simulink library "RespiratorCtrlLib"  (R2018b)
settings: Solver=VariableStepAuto  StartTime=0.0  StopTime=10.0  RelTol=1e-3
undefined symbols (not defined in the file or in its folder): AnalogMax, AnalogMin, aValveFullClose, aValveFullOpen, aValvePwm100, eSupervisorStates, fpDiffQAirInhalation, fpStatQAirInhalation, pDiffQAirAutoOffsetMax, pDiffQAirAutoOffsetMin, pDiffQAirAutoOffsetRateMax, pDiffQAirInhalationOffset, pDiffQAirScaledMax, pDiffQAirScaledMin, PressureMax, PressureMin, pStatQAirAutoOffsetMax, pStatQAirAutoOffsetMin, pStatQAirAutoOffsetRateMax, pStatQAirInhalationOffset, pStatQAirScaledMax, pStatQAirScaledMin, rPwmZeroDeg, VAnalogInputSpan, VpDiffQAirAnalogicDiagMax, VpDiffQAirAnalogicDiagMin, VpDiffQAirAnalogicMax, VpDiffQAirAnalogicMin, VpStatQAirAnalogicDiagMax, VpStatQAirAnalogicDiagMin, VpStatQAirAnalogicMax, VpStatQAirAnalogicMin
libraries: simulink x16, mbedblockslib x4, simulink_extras x2, $bdroot x2
(part 1 of 2)
settings Model: Creator=BRAUL  LastModifiedBy=VITIE

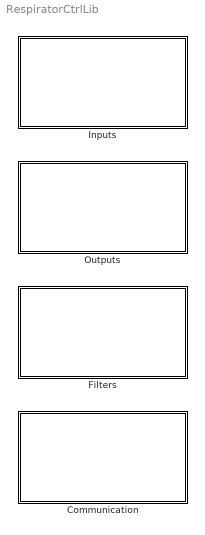
== system RespiratorCtrlLib ==
  Communication : Subsystem
  Filters : Subsystem
  Inputs : Subsystem
  Outputs : Subsystem

== system RespiratorCtrlLib/Communication ==
  Frame Multiplexer : Subsystem  TreatAsAtomicUnit=on  mask(CAN Frame multiplexer counter){MuxEndValue=1}
      mask prompts: MuxEndValue "Mutiplexer end value"
      mask help: Increase by one the output value at each sample time and reset the output (0) when previous value is equal to multiplexer end value
      settings: RTWSystemCode=Inline

== system RespiratorCtrlLib/Filters ==
  First order low pass : Subsystem  TreatAsAtomicUnit=on
      settings: RTWSystemCode=Inline
      mask Display: disp('1st Order\nLow pass')

== system RespiratorCtrlLib/Inputs ==
  Analogic Read : Subsystem  mask(Analogic Input Read){pinFunc=None, pinSelected=NC, TS=-1}
      mask prompts: pinFunc "Function"; pinSelected "Pin"; TS "Sample Time"
      mask help: Read the selected Nucleo STM32F411RE board pin as an analogic input
      mask init:
      | initAnalogicRead(gcb);
      settings: OpenFcn=|
      | setBlockPinNames(gcb);
      | open_system(gcb, 'mask');
      mask TypeOptions pinSelected: A0 | A1 | A2 | A3 | A4 | A5 | D0 | D1 | D2 | D3 | D4 | D5 | D6 | D7 | D8 | D9 | D10 | D11 | D12 | D13 | D14 | D15 | PA_0 | PA_1 | PA_2 | PA_3 | PA_4 | PA_5 | PA_6 | PA_7 | PA_8 | PA_9 | PA_10 | PA_11 | PA_12 | PA_13 | PA_14 | PA_15 | PB_0 | PB_1 | PB_2 | PB_3 | PB_4 | PB_5 | PB_6 | PB_7 | PB_8 | PB_9 | PB_10 | PB_11 | PB_12 | PB_13 | PB_14 | PB_15 | PC_0 | PC_1 | PC_2 | PC_3 | PC_4 | PC_5 | PC_6 | PC_7 | PC_8 | PC_9 | PC_10 | PC_11 | PC_12 | PC_13 | PC_14 | PC_15 | PD_2 | PH_0 | PH_1 | NC
      mask Display: disp('Analogic IN\nNone: NC')
  Button Processing : Subsystem  TreatAsAtomicUnit=on  mask(Push button debouncing){tDebounce=0.1, tSample=0.01, NDebounce=[]}
      mask prompts: tDebounce "Debounce time [sec]"; tSample "Sample time [sec]"
      mask help: Outputs the Pressed/Released state of the input push button according to user debouncing settings
      mask init:
      | % Compute debouncing sample count
      | if tSample > 0 && tDebounce > tSample
      |     
      |     NDebounce = tDebounce/tSample;
      |     
      |     maskDisplay = ['Push button\n' ...
      |                    'Debounce: ', ...
      |                    mat2str(tDebounce*1000), ...
      |                    ' ms'];
      |                
      |     set_param(gcb,'ForegroundColor', 'black');
      |     
      | else
      |     
      |     NDebounce = 2;
      |     
      |     warning([get_param(gcb, 'MaskType'), ...
      |              ' ', gcb, ' uses default debouncing setup ', ...
      |              mat2str(NDebounce), ' time steps']);
      |          
      |     maskDisplay = ['Push button\n' ...
      |                    'Debounce:\n', ...
      |                    mat2str(NDebounce), ...
      |                    ' time steps'];
      |                
      |     set_param(gcb,'ForegroundColor', 'orange');
      |     
      | end
      | 
      | % Update mask display
      | 
      | 
      | blkMask = Simulink.Mask.get(gcb);
      | blkMask.set('Display', ['disp(', char(39), maskDisplay, char(39), ')']);
      mask Display: disp('Push button\nDebounce: 100 ms')
  Differential Pressure Measurement : Subsystem  TreatAsAtomicUnit=on  mask(Differential pressure measurement){MeasName=Inhalation differential pressure, AnalogMin=VpDiffQAirAnalogicMin, AnalogMax=VpDiffQAirAnalogicMax, PressureMin=pDiffQAirScaledMin, PressureMax=pDiffQAirScaledMax, ZeroOffset=pDiffQAirInhalationOffset, CutOffFreq=fpDiffQAirInhalation, pOffsetMin=pDiffQAirAutoOffsetMin, pOffsetMax=pDiffQAirAutoOffsetMax, pOffsetRateMax=pDiffQAirAutoOffsetRateMax, VAnaMinDiag=VpDiffQAirAnalogicDiagMin, VAnaMaxDiag=VpDiffQAirAnalogicDiagMax}
      mask prompts: MeasName "Pressure name"; AnalogMin "Analogic value min [mV]"; AnalogMax "Analogic value max [mV]"; PressureMin "Pressure value min"; PressureMax "Pressure value max"; ZeroOffset "Static offset"; CutOffFreq "Filter cut-off frequency [Hz]"; pOffsetMin "Auto offset min"; pOffsetMax "Auto offset max"; pOffsetRateMax "Auto offset rate max"; VAnaMinDiag "Sensor diag analogic value min [mV]"; VAnaMaxDiag "Sensor diag analogic value max [mV]"
      mask help:
      | Convert and filter analog pressure input value to a physical measurement value using given linearization properties
      | Compute and apply a dynamic zero offset
      | Assert that sensor analogic value is contain within boundaries
      mask init:
      | % Update mask display
      | maskDisplay = [MeasName, '\nDifferential Pressure\nProcessing'];
      | 
      | blkMask = Simulink.Mask.get(gcb);
      | blkMask.set('Display', ['disp(', char(39), maskDisplay, char(39), ')']);
      mask DialogControl Container4 Prompt: ADC Conversion
      mask DialogControl Container7 Prompt: Filtering
      mask DialogControl Control3 Prompt: Pressure measurement 1st order low pass filter
      mask DialogControl Container8 Prompt: Auto Offset
      mask DialogControl Control4 Prompt: Pressure measurement dynamic auto offset
      mask DialogControl Container9 Prompt: Diagnostic
      mask DialogControl Control5 Prompt: Sensor analogic value diagnostic
      mask Display: disp('Inhalation differential pressure\nDifferential Pressure\nProcessing')
  Digital Read : Subsystem  mask(Digital Input Read){pinFunc=None, pinSelected=NC, TS=-1}
      mask prompts: pinFunc "Function"; pinSelected "Pin"; TS "Sample Time"
      mask help: Read the selected Nucleo STM32F411RE board pin as a digital input
      mask init:
      | initDigitalRead(gcb);
      settings: OpenFcn=|
      | setBlockPinNames(gcb);
      | open_system(gcb, 'mask');
      mask TypeOptions pinSelected: A0 | A1 | A2 | A3 | A4 | A5 | D0 | D1 | D2 | D3 | D4 | D5 | D6 | D7 | D8 | D9 | D10 | D11 | D12 | D13 | D14 | D15 | PA_0 | PA_1 | PA_2 | PA_3 | PA_4 | PA_5 | PA_6 | PA_7 | PA_8 | PA_9 | PA_10 | PA_11 | PA_12 | PA_13 | PA_14 | PA_15 | PB_0 | PB_1 | PB_2 | PB_3 | PB_4 | PB_5 | PB_6 | PB_7 | PB_8 | PB_9 | PB_10 | PB_11 | PB_12 | PB_13 | PB_14 | PB_15 | PC_0 | PC_1 | PC_2 | PC_3 | PC_4 | PC_5 | PC_6 | PC_7 | PC_8 | PC_9 | PC_10 | PC_11 | PC_12 | PC_13 | PC_14 | PC_15 | PD_2 | PH_0 | PH_1 | NC
      mask Display: disp('Digital IN\nNone: NC')
  Flow Computation : Subsystem  TreatAsAtomicUnit=on  mask(Flow measurement){measName=Flow, QRef=0, PStatRef=1, PDiffRef=1, kAlpha=0, kBeta=0}
      mask prompts: measName "Measurement name"; QRef "Reference flow [l/min]"; PStatRef "Reference static pressure [mbar]"; PDiffRef "Reference differential pressure [mbar]"; kAlpha "Alpha coefficient"; kBeta "Beta coefficient"
      mask help: Compute flow based on inputs static and differential pressure measurements using given parameters
      mask init:
      | % Update mask display
      | maskDisplay = [measName, '\nFlow'];
      | 
      | blkMask = Simulink.Mask.get(gcb);
      | blkMask.set('Display', ['disp(', char(39), maskDisplay, char(39), ')']);
      settings: RTWSystemCode=Inline
      mask Display: disp('Flow\nFlow')
  Input Scaling : Subsystem  TreatAsAtomicUnit=on  mask(Analog Input Scaling){inputName=MeasName, elecMin=AnalogMin, elecMax=AnalogMax, physicMin=PressureMin, physicMax=PressureMax, gain=0, offset=0}
      mask prompts: inputName "Measurement Name"; elecMin "Electrical range min [mV]"; elecMax "Electrical range max [mV]"; physicMin "Physical value min [SI]"; physicMax "Physical value max [SI]"
      mask help: Convert analog input value to a physical measurement value using given linearization properties
      mask init:
      | % Compute linearization gain & offset
      | gain = (physicMax - physicMin) / (elecMax - elecMin);
      | offset = physicMax - elecMax*gain;
      | 
      | % Update mask display
      | maskDisplay = [inputName, '\ninput\nscaling'];
      | 
      | blkMask = Simulink.Mask.get(gcb);
      | blkMask.set('Display', ['disp(', char(39), maskDisplay, char(39), ')']);
      settings: RTWSystemCode=Inline
      mask Display: disp('MeasName\ninput\nscaling')
  Static Pressure Measurement : Subsystem  TreatAsAtomicUnit=on  mask(Static pressure measurement){MeasName=Inhalation static pressure, AnalogMin=VpStatQAirAnalogicMin, AnalogMax=VpStatQAirAnalogicMax, PressureMin=pStatQAirScaledMin, PressureMax=pStatQAirScaledMax, ZeroOffset=pStatQAirInhalationOffset, CutOffFreq=fpStatQAirInhalation, VAnaMinDiag=VpStatQAirAnalogicDiagMin, VAnaMaxDiag=VpStatQAirAnalogicDiagMax}
      mask prompts: MeasName "Pressure name"; AnalogMin "Analogic value min [mV]"; AnalogMax "Analogic value max [mV]"; PressureMin "Pressure value min"; PressureMax "Pressure value max"; ZeroOffset "Static offset"; CutOffFreq "Filter cut-off frequency [Hz]"; VAnaMinDiag "Sensor diag analogic value min [mV]"; VAnaMaxDiag "Sensor diag analogic value max [mV]"
      mask help:
      | Convert and filter analog pressure input value to a physical measurement value using given linearization properties.
      | Apply a dynamic offset on the output pressure value.
      | Assert that sensor analogic value is contain within boundaries.
      mask init:
      | % Update mask display
      | maskDisplay = [MeasName, '\nStatic Pressure\nProcessing'];
      | 
      | blkMask = Simulink.Mask.get(gcb);
      | blkMask.set('Display', ['disp(', char(39), maskDisplay, char(39), ')']);
      mask DialogControl Container4 Prompt: ADC Conversion
      mask DialogControl Container7 Prompt: Filtering
      mask DialogControl Control3 Prompt: Pressure measurement 1st order low pass filter
      mask DialogControl Container9 Prompt: Diagnostic
      mask DialogControl Control5 Prompt: Sensor analogic value diagnostic
      mask Display: disp('Inhalation static pressure\nStatic Pressure\nProcessing')
  Static Pressures Offset : Subsystem  TreatAsAtomicUnit=on  mask(Static pressures offset computation){pOffsetMin=pStatQAirAutoOffsetMin, pOffsetMax=pStatQAirAutoOffsetMax, pOffsetRateMax=pStatQAirAutoOffsetRateMax}
      mask prompts: pOffsetMin "Auto offset min"; pOffsetMax "Auto offset max"; pOffsetRateMax "Auto offset rate max"
      mask help:
      | Compute pressure measurement dynamic offset of two static pressure measurements.
      | Offset is computed based on average value of inputs measurement in order to get both sensor on their mutual average value
      mask Display: disp('Static Pressures\nOffsets')
  User Setpoint : Subsystem  TreatAsAtomicUnit=on  mask(User setpoint){DefaultSetPoint=500, Increment=10, Decrement=10, MinSetPoint=300, MaxSetPoint=700}
      mask prompts: DefaultSetPoint "Default setpoint value"; Increment "Setpoint increment (on plus rising edge)"; Decrement "Setpoint decrement (on minus rising edge)"; MinSetPoint "Setpoint min value"; MaxSetPoint "Setpoint max value"
      mask help:
      | Output a user setpoint according to rising edge of 'Plus' and 'Minus' inputs.
      | When a rising edge of 'Plus' input is received, increment value is added to the previous setpoint.
      | When a rising edge of 'Minus' input is received, decrement value is substracted to the previous setpoint.
      | Final output value is saturated between setpoint min and max values.
      | When both 'Plus' and 'Minus' inputs are true at the same time, setpoint does not change.
      settings: RTWSystemCode=Inline
      mask Display:
      | port_label('input', 1, 'Plus')
      | port_label('input', 2, 'Minus')
      | port_label('output', 1, 'Setpoint')

== system RespiratorCtrlLib/Outputs ==
  Digital Write : Subsystem  mask(Digital Output Write){pinFunc=None, pinSelected=NC}
      mask prompts: pinFunc "Function"; pinSelected "Pin"
      mask help: Write the selected Nucleo STM32F411RE board pin as a digital output
      mask init:
      | initDigitalWrite(gcb);
      settings: OpenFcn=|
      | setBlockPinNames(gcb);
      | open_system(gcb, 'mask');
      mask TypeOptions pinSelected: A0 | A1 | A2 | A3 | A4 | A5 | D0 | D1 | D2 | D3 | D4 | D5 | D6 | D7 | D8 | D9 | D10 | D11 | D12 | D13 | D14 | D15 | PA_0 | PA_1 | PA_2 | PA_3 | PA_4 | PA_5 | PA_6 | PA_7 | PA_8 | PA_9 | PA_10 | PA_11 | PA_12 | PA_13 | PA_14 | PA_15 | PB_0 | PB_1 | PB_2 | PB_3 | PB_4 | PB_5 | PB_6 | PB_7 | PB_8 | PB_9 | PB_10 | PB_11 | PB_12 | PB_13 | PB_14 | PB_15 | PC_0 | PC_1 | PC_2 | PC_3 | PC_4 | PC_5 | PC_6 | PC_7 | PC_8 | PC_9 | PC_10 | PC_11 | PC_12 | PC_13 | PC_14 | PC_15 | PD_2 | PH_0 | PH_1 | NC
      mask Display: disp('Digital OUT\nNone: NC')
  PWM Output : Subsystem  mask(PWM Output Write){pinFunc=None, pinSelected=NC, pwmFreq=1000}
      mask prompts: pinFunc "Function"; pinSelected "Pin"; pwmFreq "PWM Frequency [Hz]"
      mask help: Set duty cycle, at the given frequency, of the selected Nucleo STM32F411RE board pin as a PWM output
      mask init:
      | initPwmOutput(gcb);
      settings: OpenFcn=|
      | setBlockPinNames(gcb);
      | open_system(gcb, 'mask');
      mask TypeOptions pinSelected: A0 | A1 | A2 | A3 | A4 | A5 | D0 | D1 | D2 | D3 | D4 | D5 | D6 | D7 | D8 | D9 | D10 | D11 | D12 | D13 | D14 | D15 | PA_0 | PA_1 | PA_2 | PA_3 | PA_4 | PA_5 | PA_6 | PA_7 | PA_8 | PA_9 | PA_10 | PA_11 | PA_12 | PA_13 | PA_14 | PA_15 | PB_0 | PB_1 | PB_2 | PB_3 | PB_4 | PB_5 | PB_6 | PB_7 | PB_8 | PB_9 | PB_10 | PB_11 | PB_12 | PB_13 | PB_14 | PB_15 | PC_0 | PC_1 | PC_2 | PC_3 | PC_4 | PC_5 | PC_6 | PC_7 | PC_8 | PC_9 | PC_10 | PC_11 | PC_12 | PC_13 | PC_14 | PC_15 | PD_2 | PH_0 | PH_1 | NC
      mask Display: disp('PWM OUT\nNone: NC\n1000 Hz')
  PWM Output Scaling : Subsystem  TreatAsAtomicUnit=on  mask(PWM Output Scaling){outputName=PWM, physicMin=0, physicMax=1, gain=0, offset=0}
      mask prompts: outputName "Output Name"; physicMin "Physical value min [SI]"; physicMax "Physical value max [SI]"
      mask help: Convert a physical value input to a PWM ratio between 0 and 100%
      mask init:
      | % Compute linearization gain & offset
      | gain = 100 / (physicMax - physicMin);
      | offset = 100 - physicMax*gain;
      | 
      | % Update mask display
      | maskDisplay = [outputName, '\noutput\nscaling'];
      | 
      | blkMask = Simulink.Mask.get(gcb);
      | blkMask.set('Display', ['disp(', char(39), maskDisplay, char(39), ')']);
      settings: RTWSystemCode=Inline
      mask Display: disp('PWM\noutput\nscaling')
  Valve Driver : Subsystem  TreatAsAtomicUnit=on  mask(Valve openig driver){outputName=Blower Valve, closeAngle=aValveFullClose, openAngle=aValveFullOpen, zeroDegPwm=rPwmZeroDeg, posPwmMax=aValvePwm100, gainPos=NaN, offsetPos=NaN, gainPwm=NaN, offsetPwm=0}
      mask prompts: outputName "Output Name"; closeAngle "Fully closed angle [deg]"; openAngle "Fully open angle [deg]"; zeroDegPwm "0 deg PWM [%]"; posPwmMax "Position @100% PWM [deg]"
      mask help: Convert the input opening ratio to a PWM output
      mask init:
      | % Compute opening percentage to angle target linearization gain & offset
      | gainPos = (openAngle - closeAngle)/100;
      | offsetPos = openAngle - gainPos*100;
      | 
      | % Compute position to PWM gain & offset
      | gainPwm = (100 - zeroDegPwm)/posPwmMax;
      | offsetPwm = 100 - gainPwm*posPwmMax;
      | 
      | % Update mask display
      | maskDisplay = [outputName, '\n', ...
      |                '\nClosed [0%] =', ...
      |                mat2str(closeAngle), '°\n',...
      |                'Open [100%] =', ...
      |                mat2str(openAngle), '°'];
      | 
      | blkMask = Simulink.Mask.get(gcb);
      | blkMask.set('Display', ['disp(', char(39), maskDisplay, char(39), ')']);
      settings: RTWSystemCode=Inline
      mask DialogControl grpPwmOut Prompt: PWM output
      mask Display: disp('Blower Valve\n\nClosed [0%] =-255°\nOpen [100%] =-90°')

== system RespiratorCtrlLib/Communication/Frame Multiplexer ==
  Compare To Constant : simulink/Logic and Bit Operations/Compare To Constant  relop===  const=MuxEndValue  OutDataTypeStr=boolean
  Constant : Constant  Value=0  OutDataTypeStr=uint8
  Increment Stored Integer : simulink/Additional Math & Discrete/Additional Math: Increment - Decrement/Increment Stored Integer
      settings: SourceProductName=Simulink
  Switch : Switch  Criteria=u2 ~= 0
  Unit Delay : UnitDelay  SampleTime=-1
  Mux : Outport  OutDataTypeStr=uint8
  wires:
  Compare To Constant/1 -> Switch/2
  Constant/1 -> Switch/1
  Increment Stored Integer/1 -> Switch/3
  Switch/1 -> Unit Delay/1, Mux/1
  Unit Delay/1 -> Increment Stored Integer/1, Compare To Constant/1

== system RespiratorCtrlLib/Filters/First order low pass ==
  In : Inport
  G : Inport  Port=2
  Add : Sum
  Add1 : Sum  Inputs=+-
  Product : Product
  Unit Delay : UnitDelay  SampleTime=-1
  Out : Outport
  wires:
  Add/1 -> Out/1, Unit Delay/1
  Unit Delay/1 -> Add/2, Add1/2
  In/1 -> Add1/1
  Product/1 -> Add/1
  Add1/1 -> Product/1
  G/1 -> Product/2

== system RespiratorCtrlLib/Inputs/Analogic Read ==
  Data Type Conversion : DataTypeConversion  OutDataTypeStr=single
  MBED_ANA_IN : mbedblockslib/Analog Input  Pin=2147483647  ReadResultsOnly=off  ConversionTriggerSource=Software  ExternalTriggerType=uint32( 0 )  OutputDataType=double  EnableConversionCompleteNotify=off  EnableOuputStatus=off  SampleTime=-1
      settings: SourceProductName=Simulink Coder Support Package for BBC microbit Board  SourceProductBaseCode=MICROBIT
  Out1 : Outport
  wires:
  MBED_ANA_IN/1 -> Data Type Conversion/1
  Data Type Conversion/1 -> Out1/1

== system RespiratorCtrlLib/Inputs/Button Processing ==
  BtnIn : Inport  OutDataTypeStr=boolean
  Constant : Constant  Value=NDebounce  OutDataTypeStr=uint16
  Push button debouce FSM : Stateflow chart  TreatAsAtomicUnit=on
  BtnPressed : Outport  OutDataTypeStr=boolean
  wires:
  BtnIn/1 -> Push button debouce FSM/1(BtnIn)
  Push button debouce FSM/1(BtnPressed) -> BtnPressed/1
  Constant/1 -> Push button debouce FSM/2(DebounceThd)

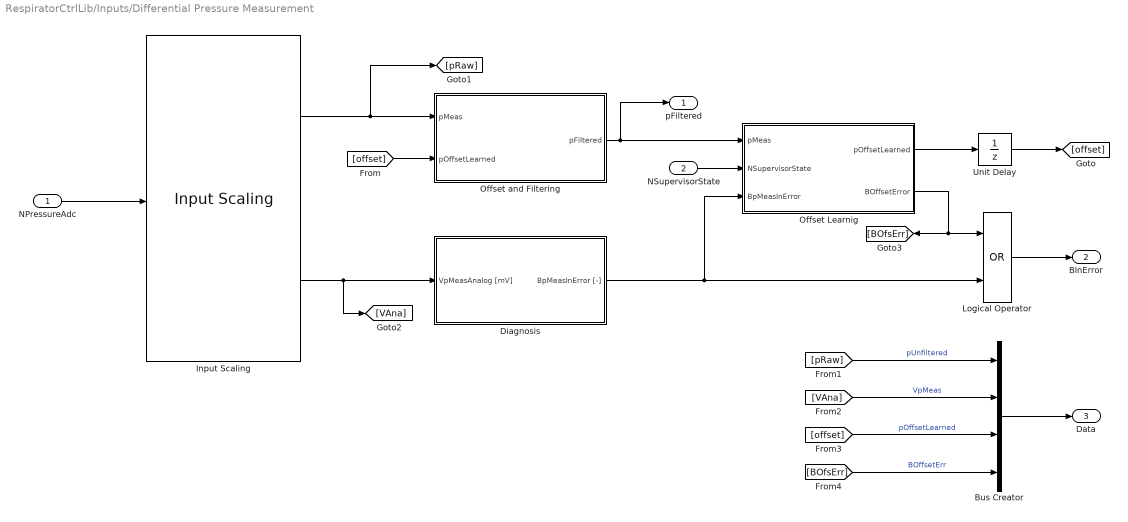
== system RespiratorCtrlLib/Inputs/Differential Pressure Measurement ==
  NPressureAdc : Inport  OutDataTypeStr=single
  NSupervisorState : Inport  Port=2  OutDataTypeStr=Enum: eSupervisorStates
  Bus Creator : BusCreator  Inputs=4  OutDataTypeStr=Bus: DiffPressureProcessingData_T
  Diagnosis : Subsystem
  Input Scaling : $bdroot/Inputs/Input Scaling  inputName=MeasName  elecMin=AnalogMin  elecMax=AnalogMax  physicMin=PressureMin  physicMax=PressureMax  gain=0  offset=0
  Logical Operator : Logic  Operator=OR  AllPortsSameDT=off  OutDataTypeStr=boolean
  Offset Learnig : Subsystem
  Offset and Filtering : Subsystem
  Unit Delay : UnitDelay  SampleTime=-1
  pFiltered : Outport
  BInError : Outport  Port=2
  Data : Outport  Port=3  OutDataTypeStr=Bus: DiffPressureProcessingData_T
  wires:
  [BOfsErr] -> Bus Creator/4  "BOffsetErr"
  [VAna] -> Bus Creator/2  "VpMeas"
  [offset] -> Bus Creator/3  "pOffsetLearned"
  [pRaw] -> Bus Creator/1  "pUnfiltered"
  NPressureAdc/1 -> Input Scaling/1
  Input Scaling/2 -> [VAna], Diagnosis/1(VpMeasAnalog [mV])
  Input Scaling/1 -> [pRaw], Offset and Filtering/1(pMeas)
  Offset and Filtering/1(pFiltered) -> Offset Learnig/1(pMeas), pFiltered/1
  NSupervisorState/1 -> Offset Learnig/2(NSupervisorState)
  Offset Learnig/2(BOffsetError) -> Logical Operator/1, [BOfsErr]
  Diagnosis/1(BpMeasInError [-]) -> Offset Learnig/3(BpMeasInError), Logical Operator/2
  Logical Operator/1 -> BInError/1
  Offset Learnig/1(pOffsetLearned) -> Unit Delay/1
  Unit Delay/1 -> [offset]
  [offset] -> Offset and Filtering/2(pOffsetLearned)
  Bus Creator/1 -> Data/1

== system RespiratorCtrlLib/Inputs/Digital Read ==
  Data Type Conversion : DataTypeConversion  OutDataTypeStr=boolean
  MBED_DIG_IN : mbedblockslib/Digital Read  Pin=2147483647  Direction=input  SampleTime=-1
      settings: SourceProductName=Simulink Coder Support Package for BBC microbit Board  SourceProductBaseCode=MICROBIT
  Out1 : Outport
  wires:
  MBED_DIG_IN/1 -> Data Type Conversion/1
  Data Type Conversion/1 -> Out1/1

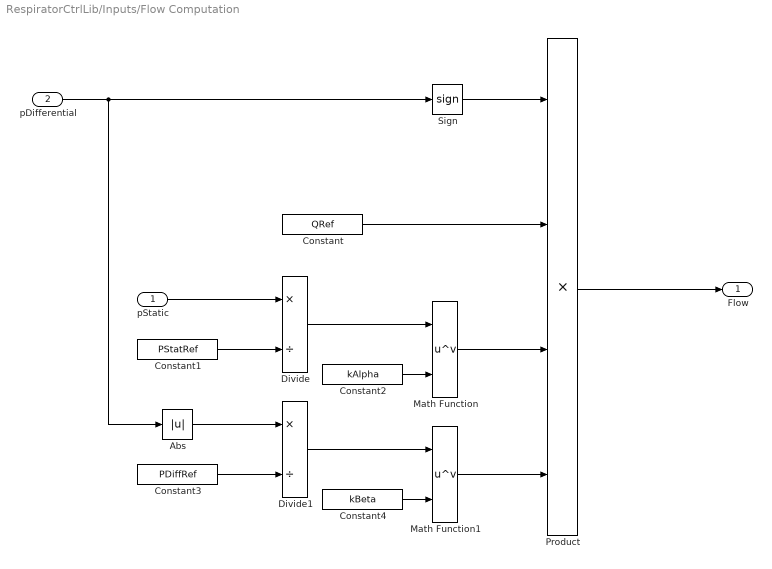
== system RespiratorCtrlLib/Inputs/Flow Computation ==
  pStatic : Inport  OutDataTypeStr=single  Unit=mbar  PortDimensions=1
  pDifferential : Inport  Port=2  OutDataTypeStr=single  Unit=mbar  PortDimensions=1
  Abs : Abs
  Constant : Constant  Value=QRef
  Constant1 : Constant  Value=PStatRef
  Constant2 : Constant  Value=kAlpha
  Constant3 : Constant  Value=PDiffRef
  Constant4 : Constant  Value=kBeta
  Divide : Product  Inputs=*/
  Divide1 : Product  Inputs=*/
  Math Function : Math  Operator=pow  SaturateOnIntegerOverflow=on
  Math Function1 : Math  Operator=pow  SaturateOnIntegerOverflow=on
  Product : Product  Inputs=4
  Sign : Signum
  Flow : Outport  OutDataTypeStr=single  Unit=l/min  PortDimensions=1
  wires:
  Product/1 -> Flow/1
  pDifferential/1 -> Abs/1, Sign/1
  Sign/1 -> Product/1
  Constant/1 -> Product/2
  pStatic/1 -> Divide/1
  Constant1/1 -> Divide/2
  Divide/1 -> Math Function/1
  Constant2/1 -> Math Function/2
  Math Function/1 -> Product/3
  Constant4/1 -> Math Function1/2
  Math Function1/1 -> Product/4
  Divide1/1 -> Math Function1/1
  Constant3/1 -> Divide1/2
  Abs/1 -> Divide1/1

== system RespiratorCtrlLib/Inputs/Input Scaling ==
  NInputRaw : Inport
  Add : Sum
  Constant2 : Constant  Value=offset  OutDataTypeStr=single
  Gain : Gain  Gain=gain
  Gain1 : Gain  Gain=VAnalogInputSpan
      settings: AttributesFormatString=%<Gain>
  NInputPhysic : Outport
  VInputAnalog : Outport  Port=2
  wires:
  Gain1/1 -> Gain/1, VInputAnalog/1
  Add/1 -> NInputPhysic/1
  Constant2/1 -> Add/2
  Gain/1 -> Add/1
  NInputRaw/1 -> Gain1/1

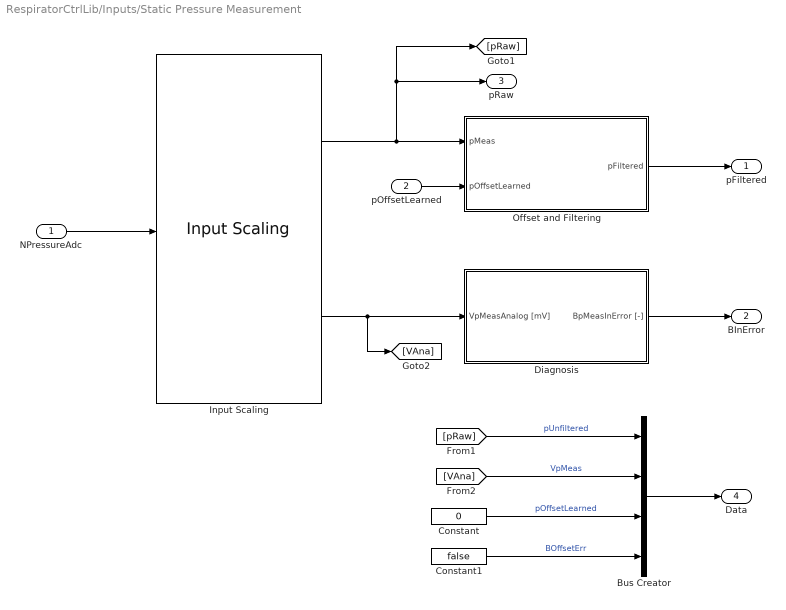
== system RespiratorCtrlLib/Inputs/Static Pressure Measurement ==
  NPressureAdc : Inport  OutDataTypeStr=single
  pOffsetLearned : Inport  Port=2  OutDataTypeStr=single
  Bus Creator : BusCreator  Inputs=4  OutDataTypeStr=Bus: DiffPressureProcessingData_T
  Constant : Constant  Value=0  OutDataTypeStr=single
  Constant1 : Constant  Value=false  OutDataTypeStr=boolean
  Diagnosis : Subsystem
  Input Scaling : $bdroot/Inputs/Input Scaling  inputName=MeasName  elecMin=AnalogMin  elecMax=AnalogMax  physicMin=PressureMin  physicMax=PressureMax  gain=0  offset=0
  Offset and Filtering : Subsystem
  pFiltered : Outport
  BInError : Outport  Port=2
  pRaw : Outport  Port=3
  Data : Outport  Port=4  OutDataTypeStr=Bus: DiffPressureProcessingData_T
  wires:
  Constant1/1 -> Bus Creator/4  "BOffsetErr"
  Bus Creator/1 -> Data/1
  pOffsetLearned/1 -> Offset and Filtering/2(pOffsetLearned)
  Diagnosis/1(BpMeasInError [-]) -> BInError/1
  Offset and Filtering/1(pFiltered) -> pFiltered/1
  Input Scaling/1 -> Offset and Filtering/1(pMeas), [pRaw], pRaw/1
  Input Scaling/2 -> Diagnosis/1(VpMeasAnalog [mV]), [VAna]
  NPressureAdc/1 -> Input Scaling/1
  [pRaw] -> Bus Creator/1  "pUnfiltered"
  Constant/1 -> Bus Creator/3  "pOffsetLearned"
  [VAna] -> Bus Creator/2  "VpMeas"

== system RespiratorCtrlLib/Inputs/Static Pressures Offset ==
  pStat1Raw : Inport  OutDataTypeStr=single
  pStat2Raw : Inport  Port=2  OutDataTypeStr=single
  pStat1 : Inport  Port=3  OutDataTypeStr=single
  pStat2 : Inport  Port=4  OutDataTypeStr=single
  Bp1InError : Inport  Port=5  OutDataTypeStr=boolean
  Bp2InError : Inport  Port=6  OutDataTypeStr=boolean
  NSupervisorState : Inport  Port=7  OutDataTypeStr=Enum: eSupervisorStates
  Compare To Constant1 : simulink/Logic and Bit Operations/Compare To Constant  relop===  const=eSupervisorStates.NRespiratorInit  OutDataTypeStr=boolean
  Pressure offset computation : Subsystem
  p1OffsetLearned : Outport  InitialOutput=0
  p2OffsetLearned : Outport  Port=2  InitialOutput=0
  Bp1OffsetError : Outport  Port=3  OutDataTypeStr=boolean  InitialOutput=false
  Bp2OffsetError : Outport  Port=4  OutDataTypeStr=boolean  InitialOutput=false
  wires:
  pStat2Raw/1 -> Pressure offset computation/2(pStat2Raw)
  pStat1Raw/1 -> Pressure offset computation/1(pStat1Raw)
  NSupervisorState/1 -> Compare To Constant1/1
  Compare To Constant1/1 -> Pressure offset computation/Enable
  pStat1/1 -> Pressure offset computation/3(pStat1)
  pStat2/1 -> Pressure offset computation/4(pStat2)
  Bp1InError/1 -> Pressure offset computation/5(Bp1InError)
  Bp2InError/1 -> Pressure offset computation/6(Bp2InError)
  Pressure offset computation/1(p1OffsetLearned) -> p1OffsetLearned/1
  Pressure offset computation/2(p2OffsetLearned) -> p2OffsetLearned/1
  Pressure offset computation/3(Bp1OffsetError) -> Bp1OffsetError/1
  Pressure offset computation/4(Bp2OffsetError) -> Bp2OffsetError/1

== system RespiratorCtrlLib/Inputs/User Setpoint ==
  PlusBtn : Inport  OutDataTypeStr=boolean  PortDimensions=1
  MinusBtn : Inport  Port=2  OutDataTypeStr=boolean  PortDimensions=1
  Detect Increase : simulink/Logic and Bit Operations/Detect Increase  vinit=0.0  OutDataTypeStr=boolean
  Detect Increase1 : simulink/Logic and Bit Operations/Detect Increase  vinit=0.0  OutDataTypeStr=boolean
  Logical Operator : Logic  Operator=XOR  AllPortsSameDT=off  OutDataTypeStr=boolean
  Subsystem : Subsystem
  Setpoint : Outport  OutDataTypeStr=single  PortDimensions=1
  wires:
  Detect Increase1/1 -> Subsystem/2(MinusBtn)
  Detect Increase/1 -> Subsystem/1(PlusBtn)
  MinusBtn/1 -> Logical Operator/2, Detect Increase1/1
  PlusBtn/1 -> Logical Operator/1, Detect Increase/1
  Logical Operator/1 -> Subsystem/Trigger
  Subsystem/1(Setpoint) -> Setpoint/1

== system RespiratorCtrlLib/Outputs/Digital Write ==
  In1 : Inport
  Detect Change : simulink/Logic and Bit Operations/Detect Change  vinit=0  OutDataTypeStr=boolean
  Set on value changed : Subsystem
  wires:
  In1/1 -> Detect Change/1, Set on value changed/1(In1)
  Detect Change/1 -> Set on value changed/Enable

== system RespiratorCtrlLib/Outputs/PWM Output ==
  In1 : Inport
  Detect Change : simulink/Logic and Bit Operations/Detect Change  vinit=0  OutDataTypeStr=boolean
  Set on value changed : Subsystem
  wires:
  In1/1 -> Detect Change/1, Set on value changed/1(In1)
  Detect Change/1 -> Set on value changed/Enable

== system RespiratorCtrlLib/Outputs/PWM Output Scaling ==
  NPhysicTgt : Inport
  Add : Sum
  Constant2 : Constant  Value=offset
  Gain : Gain  Gain=gain
  Saturation : Saturate  UpperLimit=100  LowerLimit=0
  rPwmOut : Outport
  wires:
  Saturation/1 -> rPwmOut/1
  NPhysicTgt/1 -> Gain/1
  Gain/1 -> Add/1
  Constant2/1 -> Add/2
  Add/1 -> Saturation/1

== system RespiratorCtrlLib/Outputs/Valve Driver ==
  rOpeningTgt : Inport
  Add : Sum
  Add1 : Sum
  Constant1 : Constant  Value=offsetPwm  OutDataTypeStr=single
  Constant2 : Constant  Value=offsetPos  OutDataTypeStr=single
  Gain : Gain  Gain=gainPos  OutDataTypeStr=single
  Gain2 : Gain  Gain=gainPwm  OutDataTypeStr=single
  Saturation : Saturate  UpperLimit=100  LowerLimit=zeroDegPwm
  rPwmOut : Outport
  aPosTgt : Outport  Port=2  OutDataTypeStr=single
  wires:
  Add1/1 -> Saturation/1
  Gain2/1 -> Add1/1
  Constant1/1 -> Add1/2
  Add/1 -> Gain2/1, aPosTgt/1
  Saturation/1 -> rPwmOut/1
  rOpeningTgt/1 -> Gain/1
  Gain/1 -> Add/1
  Constant2/1 -> Add/2

== system RespiratorCtrlLib/Inputs/Differential Pressure Measurement/Diagnosis ==
  VpMeasAnalog [mV] : Inport
  Constant : Constant  Value=VAnaMinDiag  OutDataTypeStr=single
  Constant1 : Constant  Value=VAnaMaxDiag  OutDataTypeStr=single
  Constant2 : Constant  Value=0  OutDataTypeStr=boolean
  Constant3 : Constant  Value=25  OutDataTypeStr=single
  Constant4 : Constant  Value=10  OutDataTypeStr=single
  Failure Counter : Subsystem  TreatAsAtomicUnit=on  mask(Failure Counter){temp=off, TSample=10, ena=off}
      mask prompts: temp "Is Temporal?"; TSample "Sample Time (ms)"; ena "Need to be Enable?"
      mask init:
      | %Find inputs to change name
      | rInc=find_system(gcbh,'LookUnderMasks','all','FollowLinks','on','RegExp','on','Name','rInc');
      | rDec=find_system(gcbh,'LookUnderMasks','all','FollowLinks','on','RegExp','on','Name','rDec');
      | rFail=find_system(gcbh,'LookUnderMasks','all','FollowLinks','on','RegExp','on','Name','rFail');
      | % Active enable
      | ena_block=find_system(gcbh,'LookUnderMasks','all','FollowLinks','on','Name','enable');
      | if ena && isempty(ena_block)  
      |     add_block('simulink/Ports & Subsystems/Enable',[gcb,'/enable'])
      | elseif not(ena) && not(isempty(ena_block))
      |     delete_block([gcb,'/enable']);
      | end
      | 
      | %Verify if Temporal or not
      | if temp
      |     set_param([gcb '/Sample'],'Value',mat2str(eval(TSample)))
      |     %sample=replace_block(gcbh,'Name','Sample','GDElib_functions/SampleTime','noprompt');
      |     %set_param(gcb,'DataType','single','TSample',mat2str(eval(TSample)/1000));
      |     set_param(rInc,'Name','rInc [%/ms]')
      |     set_param(rDec,'Name','rDec [%/ms]')
      |     set_param(rFail,'Name','rFailureCounter [%]')
      |     status=['Temporal \n' TSample ' ms'];
      | else
      |     set_param([gcb,'/Sample'],'Value','1');
      |     set_param(rInc,'Name','rInc [%/cp]')
      |     set_param(rDec,'Name','rDec [%/cp]')
      |     set_param(rFail,'Name','rFailureCounter [%]')
      |     status='Not Temporal';
      |     
      | end
      settings: AttributesFormatString=%<StaticLinkStatus>
      mask Callback temp:
      | maskedit_FailC=get_param(gcb,'temp');
      | vis_FailC = get_param(gcb, 'maskvisibilities');
      | vis_FailC{2} = maskedit_FailC;
      | set_param(gcb,'maskvisibilities',vis_FailC);
      | clear vis_FailC maskedit_FailC;
      mask TypeOptions TSample: 1 | 2 | 5 | 10 | 20 | 50 | 100 | 1000
      mask Display: disp(status)
  Logical Operator : Logic  Operator=OR  AllPortsSameDT=off  OutDataTypeStr=boolean
  RawMax : RelationalOperator  Operator=>  RndMeth=Nearest  InputSameDT=on
  RawMax1 : RelationalOperator  Operator=<  RndMeth=Nearest  InputSameDT=on
  Terminator : Terminator
  BpMeasInError [-] : Outport
  wires:
  Constant1/1 -> RawMax/2
  Constant/1 -> RawMax1/2
  Constant4/1 -> Failure Counter/3(rDec [%/cp])
  Constant3/1 -> Failure Counter/2(rInc [%/cp])
  Constant2/1 -> Failure Counter/4(BReset [-])
  RawMax/1 -> Logical Operator/1
  RawMax1/1 -> Logical Operator/2
  Logical Operator/1 -> Failure Counter/1(BDetectedFailure)
  Failure Counter/2(rFailureCounter [%]) -> Terminator/1
  VpMeasAnalog [mV]/1 -> RawMax/1, RawMax1/1
  Failure Counter/1(BConfirmedFailure) -> BpMeasInError [-]/1

== system RespiratorCtrlLib/Inputs/Differential Pressure Measurement/Offset Learnig ==
  pMeas : Inport
  NSupervisorState : Inport  Port=2  OutDataTypeStr=Enum: eSupervisorStates
  BpMeasInError : Inport  Port=3
  Compare To Constant1 : simulink/Logic and Bit Operations/Compare To Constant  relop===  const=eSupervisorStates.NRespiratorInit  OutDataTypeStr=boolean
  Pressure offset computation : Subsystem
  pOffsetLearned : Outport
  BOffsetError : Outport  Port=2
  wires:
  Compare To Constant1/1 -> Pressure offset computation/Enable
  NSupervisorState/1 -> Compare To Constant1/1
  pMeas/1 -> Pressure offset computation/1(pMeas)
  Pressure offset computation/1(pOffsetLearned) -> pOffsetLearned/1
  Pressure offset computation/2(BOffsetError) -> BOffsetError/1
  BpMeasInError/1 -> Pressure offset computation/2(BpMeasInError)

== system RespiratorCtrlLib/Inputs/Differential Pressure Measurement/Offset and Filtering ==
  pMeas : Inport
  pOffsetLearned : Inport  Port=2
  Add : Sum  Inputs=++-
  Constant : Constant  Value=CutOffFreq  OutDataTypeStr=single
  Constant1 : Constant  Value=ZeroOffset  OutDataTypeStr=single
  Constant2 : Constant  Value=false  OutDataTypeStr=boolean
  Filtre_1er_ordre_Init : Subsystem  mask(FIRST ORDER FILTER INIT){TaskTime=SYNC, InType=Frequency}
      mask prompts: TaskTime "Task Execution Time"; InType "Filter Input Type :"
      mask help:
      | This block is a first-order filter with the following equation :
      | If f*Te< 0.5 with f=1(2*Pi*TAU)
      | y(k)=1/[1+Te/Tau]*y(k-1) + Te/Tau/[1+Te/Tau]*u(k).
      | Else y(k)=u(k)
      | In case of Reset, the output is initialized to INIT value.
      | In case of permanent reset, y(k)= INIT.
      mask init:
      | x=[-5:0.5:5];
      | y=1-exp(-(x+5)/1);
      | 
      | %get the mask level block path
      | blockPath=gcb;
      | 
      | %get the first inport and rename it depending on the value type selected by the user
      | Inports.Path=find_system(blockPath,'SearchDepth',1,'FollowLinks','on','regexp','on','LookUnderMasks','on','BlockType','Inport');
      | Inports.Handle=get_param(Inports.Path,'Handle');
      | Inports.Number=get_param(Inports.Path,'Port');
      | 
      | for i=1:1:length(Inports.Number)
      |     if strcmp(Inports.Number(i,1),'1')
      |         if strcmp(InType,'Tau')
      |             set_param(Inports.Handle{i,1},'Name','Tau [s]')
      |         else
      |             set_param(Inports.Handle{i,1},'Name','Frequency [Hz]')
      |         end
      |     end
      | end
      | 
      | Inports2.Path=find_system([blockPath '/Coefficients'],'SearchDepth',1,'FollowLinks','on','regexp','on','LookUnderMasks','on','BlockType','Inport');
      | Inports2.Handle=get_param(Inports2.Path,'Handle');
      | Inports2.Number=get_param(Inports2.Path,'Port');
      | 
      | for i=1:1:length(Inports2.Number)
      |     if strcmp(Inports2.Number(i,1),'1')
      |         if strcmp(InType,'Tau')
      |             set_param(Inports2.Handle{i,1},'Name','Tau [s]')
      |         else
      |             set_param(Inports2.Handle{i,1},'Name','Frequency [Hz]')
      |         end
      |     end
      | end
      | 
      | %find all constants
      | Constant.Path=find_system(blockPath,'SearchDepth',2,'FollowLinks','on','regexp','on','LookUnderMasks','on','BlockType','Constant');
      | Constant.Name=get_param(Constant.Path,'Name');
      | 
      | for i=1:1:length(Constant.Name(:,1))
      |     %set the constants for the selection Tau / frequency
      |     if strcmp(Constant.Name{i,1},'FilterInputTypeSelector')
      |         if strcmp(InType,'Frequency')
      |             set_param(Constant.Path{i,1},'Value','0')
      |         elseif strcmp(InType,'Tau')
      |             set_param(Constant.Path{i,1},'Value','1')
      |         end
      |     end
      | 
      |     %set the constants for the selection synchronous/asynchronous task time
      |     if strcmp(Constant.Name{i,1},'TaskTimeTypeSelector')
      |         if strcmp(TaskTime,'SYNC')
      |             set_param(Constant.Path{i,1},'Value','0')
      |         else
      |             set_param(Constant.Path{i,1},'Value','1')
      |         end
      |     end
      |     
      |     %set the constant for the task time
      |     if strcmp(Constant.Name{i,1},'Time') && ~strcmp(TaskTime,'SYNC')
      |         set_param(Constant.Path{i,1},'Value',num2str(str2double(regexprep(TaskTime,'ms',''))/1000))
      |     end
      | end
      mask Help:
      | This block is a first-order filter with the following equation :
      | If f*Te< 0.5 with f=1(2*Pi*TAU)
      | y(k)=1/[1+Te/Tau]*y(k-1) + Te/Tau/[1+Te/Tau]*u(k).
      | Else y(k)=u(k)
      | In case of Reset, the output is initialized to INIT value.
      | In case of permanent reset, y(k)= INIT.
      mask TypeOptions TaskTime: 1ms | 2ms | 5ms | 10ms | 20ms | 50ms | 100ms | 1000ms | SYNC
      mask TypeOptions InType: Tau | Frequency
      mask Display:
      | plot(x,y);
      | plot([min(x),max(x),NaN],[0,0,NaN]);
      | plot(min(-1,min(x)*1.5),min(-1,min(y)*1.5),max(1,max(x)*1.5),max(1,max(y)*1.5));
      | text(min(-0.9,min(x)*1.2),min(-0.9,min(y)*1.2),'First-Order Filter Init');
      | disp(['' TaskTime ''])% ] Cylinders \n Input Size : ' num2str(NTot)])
  pFiltered : Outport
  wires:
  Constant/1 -> Filtre_1er_ordre_Init/1(Frequency [Hz])
  Add/1 -> Filtre_1er_ordre_Init/3(INIT), Filtre_1er_ordre_Init/2(INPUT)
  pMeas/1 -> Add/1
  Constant1/1 -> Add/2
  pOffsetLearned/1 -> Add/3
  Constant2/1 -> Filtre_1er_ordre_Init/4(RESET)
  Filtre_1er_ordre_Init/1(OUTPUT) -> pFiltered/1

== system RespiratorCtrlLib/Inputs/Static Pressure Measurement/Diagnosis ==
  VpMeasAnalog [mV] : Inport
  Constant : Constant  Value=VAnaMinDiag  OutDataTypeStr=single
  Constant1 : Constant  Value=VAnaMaxDiag  OutDataTypeStr=single
  Constant2 : Constant  Value=0  OutDataTypeStr=boolean
  Constant3 : Constant  Value=25  OutDataTypeStr=single
  Constant4 : Constant  Value=10  OutDataTypeStr=single
  Failure Counter : Subsystem  TreatAsAtomicUnit=on  mask(Failure Counter){temp=off, TSample=10, ena=off}
      mask prompts: temp "Is Temporal?"; TSample "Sample Time (ms)"; ena "Need to be Enable?"
      mask init: same as RespiratorCtrlLib/Inputs/Differential Pressure Measurement/Diagnosis/Failure Counter
      settings: AttributesFormatString=%<StaticLinkStatus>
      mask Callback temp:
      | maskedit_FailC=get_param(gcb,'temp');
      | vis_FailC = get_param(gcb, 'maskvisibilities');
      | vis_FailC{2} = maskedit_FailC;
      | set_param(gcb,'maskvisibilities',vis_FailC);
      | clear vis_FailC maskedit_FailC;
      mask TypeOptions TSample: 1 | 2 | 5 | 10 | 20 | 50 | 100 | 1000
      mask Display: disp(status)
  Logical Operator : Logic  Operator=OR  AllPortsSameDT=off  OutDataTypeStr=boolean
  RawMax : RelationalOperator  Operator=>  RndMeth=Nearest  InputSameDT=on
  RawMax1 : RelationalOperator  Operator=<  RndMeth=Nearest  InputSameDT=on
  Terminator : Terminator
  BpMeasInError [-] : Outport
  wires:
  Failure Counter/1(BConfirmedFailure) -> BpMeasInError [-]/1
  VpMeasAnalog [mV]/1 -> RawMax1/1, RawMax/1
  Failure Counter/2(rFailureCounter [%]) -> Terminator/1
  Logical Operator/1 -> Failure Counter/1(BDetectedFailure)
  RawMax1/1 -> Logical Operator/2
  RawMax/1 -> Logical Operator/1
  Constant2/1 -> Failure Counter/4(BReset [-])
  Constant3/1 -> Failure Counter/2(rInc [%/cp])
  Constant4/1 -> Failure Counter/3(rDec [%/cp])
  Constant/1 -> RawMax1/2
  Constant1/1 -> RawMax/2

== system RespiratorCtrlLib/Inputs/Static Pressure Measurement/Offset and Filtering ==
  pMeas : Inport
  pOffsetLearned : Inport  Port=2
  Add : Sum  Inputs=++-
  Constant : Constant  Value=CutOffFreq  OutDataTypeStr=single
  Constant1 : Constant  Value=ZeroOffset  OutDataTypeStr=single
  Constant2 : Constant  Value=false  OutDataTypeStr=boolean
  Filtre_1er_ordre_Init : Subsystem  mask(FIRST ORDER FILTER INIT){TaskTime=SYNC, InType=Frequency}
      mask prompts: TaskTime "Task Execution Time"; InType "Filter Input Type :"
      mask help:
      | This block is a first-order filter with the following equation :
      | If f*Te< 0.5 with f=1(2*Pi*TAU)
      | y(k)=1/[1+Te/Tau]*y(k-1) + Te/Tau/[1+Te/Tau]*u(k).
      | Else y(k)=u(k)
      | In case of Reset, the output is initialized to INIT value.
      | In case of permanent reset, y(k)= INIT.
      mask init: same as RespiratorCtrlLib/Inputs/Differential Pressure Measurement/Offset and Filtering/Filtre_1er_ordre_Init
      mask Help:
      | This block is a first-order filter with the following equation :
      | If f*Te< 0.5 with f=1(2*Pi*TAU)
      | y(k)=1/[1+Te/Tau]*y(k-1) + Te/Tau/[1+Te/Tau]*u(k).
      | Else y(k)=u(k)
      | In case of Reset, the output is initialized to INIT value.
      | In case of permanent reset, y(k)= INIT.
      mask TypeOptions TaskTime: 1ms | 2ms | 5ms | 10ms | 20ms | 50ms | 100ms | 1000ms | SYNC
      mask TypeOptions InType: Tau | Frequency
      mask Display:
      | plot(x,y);
      | plot([min(x),max(x),NaN],[0,0,NaN]);
      | plot(min(-1,min(x)*1.5),min(-1,min(y)*1.5),max(1,max(x)*1.5),max(1,max(y)*1.5));
      | text(min(-0.9,min(x)*1.2),min(-0.9,min(y)*1.2),'First-Order Filter Init');
      | disp(['' TaskTime ''])% ] Cylinders \n Input Size : ' num2str(NTot)])
  pFiltered : Outport
  wires:
  Filtre_1er_ordre_Init/1(OUTPUT) -> pFiltered/1
  Constant2/1 -> Filtre_1er_ordre_Init/4(RESET)
  pOffsetLearned/1 -> Add/3
  Constant1/1 -> Add/2
  pMeas/1 -> Add/1
  Add/1 -> Filtre_1er_ordre_Init/2(INPUT), Filtre_1er_ordre_Init/3(INIT)
  Constant/1 -> Filtre_1er_ordre_Init/1(Frequency [Hz])

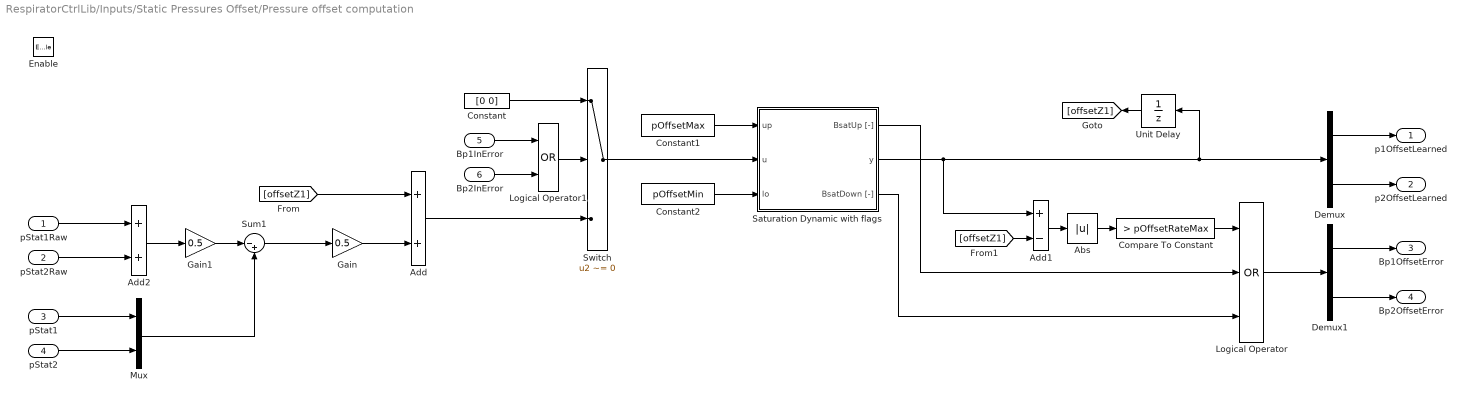
== system RespiratorCtrlLib/Inputs/Static Pressures Offset/Pressure offset computation ==
  pStat1Raw : Inport  OutDataTypeStr=single
  pStat2Raw : Inport  Port=2  OutDataTypeStr=single
  pStat1 : Inport  Port=3  OutDataTypeStr=single
  pStat2 : Inport  Port=4  OutDataTypeStr=single
  Bp1InError : Inport  Port=5  OutDataTypeStr=boolean
  Bp2InError : Inport  Port=6  OutDataTypeStr=boolean
  Enable : EnablePort  StatesWhenEnabling=reset
  Abs : Abs
  Add : Sum
  Add1 : Sum  Inputs=+-
  Add2 : Sum
  Compare To Constant : simulink/Logic and Bit Operations/Compare To Constant  relop=>  const=pOffsetRateMax  OutDataTypeStr=boolean
  Constant : Constant  Value=[0 0]  OutDataTypeStr=single
  Constant1 : Constant  Value=pOffsetMax  OutDataTypeStr=single
  Constant2 : Constant  Value=pOffsetMin  OutDataTypeStr=single
  Demux : Demux  Outputs=2
  Demux1 : Demux  Outputs=2
  Gain : Gain  Gain=0.5
  Gain1 : Gain  Gain=0.5
  Logical Operator : Logic  Operator=OR  Inputs=3  AllPortsSameDT=off  OutDataTypeStr=boolean
  Logical Operator1 : Logic  Operator=OR  AllPortsSameDT=off  OutDataTypeStr=boolean
  Mux : Mux  Inputs=2
  Saturation Dynamic with flags : Subsystem  mask(Saturation Dynamic){OutMin=[], OutMax=[], OutDataTypeStr=Inherit: Same as second input, OutputDataTypeScalingMode=Same as second input, OutDataType=fixdt(1, 16), OutScaling=2^-10, LockScale=off, RndMeth=Floor, DoSatur=off}
      mask prompts: OutMin "Output minimum:"; OutMax "Output maximum:"; OutDataTypeStr "Output data type:"; OutputDataTypeScalingMode "Output data type mode:"; OutDataType "Output data type (e.g. fixdt(1, 16), fixdt('single')):"; OutScaling "Output scaling (Slope, e.g. 2^-9 or [Slope Bias], e.g. [1.25 3]):"; LockScale "Lock output data type setting against changes by the fixed-point tools"; RndMeth "Integer rounding mode:"; DoSatur "Saturate on integer overflow"
      mask help: Bound the range of the second input by using the first input (upper limit) and the third input (lower limit).
      mask init:
      | blkH = gcbh;
      | blkName = getfullname(blkH);
      | 
      | switch_blks = {'Switch','Switch2'}; 
      | for i = 1:length(switch_blks)
      |   set_param([blkName,'/',switch_blks{i}], ...
      |       'RndMeth', RndMeth, ...
      | 	  'DoSatur', DoSatur);
      | end
      | 
      | propBlk = [blkName, '/Data Type Propagation'];
      | 
      | if strcmp(OutputDataTypeScalingMode, 'Same as second input')
      |     set_param(propBlk, 'PropDataTypeMode', 'Inherit via propagation rule', ...
      |                        'PropScalingMode',  'Inherit via propagation rule');
      | else
      |     scaling = OutScaling;
      |     switch OutputDataTypeScalingMode
      |       case 'double'
      |         dataType = 'fixdt(''double'')';
      |       case 'single'
      |         dataType = 'fixdt(''single'')';
      |       case 'int8'
      |         dataType = 'fixdt(1,8,0)';
      |       case 'uint8'
      |         dataType = 'fixdt(0,8,0)';
      |       case 'int16'
      |         dataType = 'fixdt(1,16,0)';
      |       case 'uint16'
      |         dataType = 'fixdt(0,16,0)';
      |       case 'int32'
      |         dataType = 'fixdt(1,32,0)';
      |       case 'uint32'
      |         dataType = 'fixdt(0,32,0)';
      |       case 'Specify via dialog'
      |         dataType = OutDataType;
      |     end
      |     
      |     set_param(propBlk, 'PropDataTypeMode', 'Specify via dialog', ...
      |                        'PropScalingMode',  'Specify via dialog', ...
      |                        'PropDataType',     dataType, ...
      |                        'PropScaling',      scaling);
      | end
      mask Callback OutDataTypeStr: fixptdialog(gcbh)
      mask TypeOptions OutputDataTypeScalingMode: double | single | int8 | uint8 | int16 | uint16 | int32 | uint32 | Specify via dialog | Same as second input
      mask Callback OutputDataTypeScalingMode: fixptdialog(gcbh)
      mask Callback OutDataType: fixptdialog(gcbh)
      mask TypeOptions RndMeth: Ceiling | Convergent | Floor | Nearest | Round | Simplest | Zero
      mask Display: plot([0.15 0.85],[.5 .5],[.5 .5],[0.05 0.95],0.15+0.7*[0 .25 .75 1],0.05+0.9*[.25 .25 .75 .75]);
  Sum1 : Sum  Inputs=|-+
  Switch : Switch  Criteria=u2 ~= 0
  Unit Delay : UnitDelay  SampleTime=-1
  p1OffsetLearned : Outport  InitialOutput=0
  p2OffsetLearned : Outport  Port=2  InitialOutput=0
  Bp1OffsetError : Outport  Port=3  OutDataTypeStr=boolean  InitialOutput=false
  Bp2OffsetError : Outport  Port=4  OutDataTypeStr=boolean  InitialOutput=false
  wires:
  pStat2Raw/1 -> Add2/2
  pStat1Raw/1 -> Add2/1
  Logical Operator1/1 -> Switch/2
  Constant/1 -> Switch/1
  Unit Delay/1 -> [offsetZ1]
  Gain/1 -> Add/2
  [offsetZ1] -> Add/1
  Add/1 -> Switch/3
  Switch/1 -> Saturation Dynamic with flags/2(u)
  Saturation Dynamic with flags/2(y) -> Unit Delay/1, Demux/1, Add1/1
  Constant1/1 -> Saturation Dynamic with flags/1(up)
  Constant2/1 -> Saturation Dynamic with flags/3(lo)
  [offsetZ1] -> Add1/2
  Add1/1 -> Abs/1
  Abs/1 -> Compare To Constant/1
  Compare To Constant/1 -> Logical Operator/1
  Saturation Dynamic with flags/1(BsatUp [-]) -> Logical Operator/2
  Saturation Dynamic with flags/3(BsatDown [-]) -> Logical Operator/3
  Bp1InError/1 -> Logical Operator1/1
  Bp2InError/1 -> Logical Operator1/2
  pStat1/1 -> Mux/1
  pStat2/1 -> Mux/2
  Add2/1 -> Gain1/1
  Gain1/1 -> Sum1/1
  Mux/1 -> Sum1/2
  Sum1/1 -> Gain/1
  Logical Operator/1 -> Demux1/1
  Demux/1 -> p1OffsetLearned/1
  Demux/2 -> p2OffsetLearned/1
  Demux1/1 -> Bp1OffsetError/1
  Demux1/2 -> Bp2OffsetError/1

== system RespiratorCtrlLib/Inputs/User Setpoint/Subsystem ==
  PlusBtn : Inport  OutDataTypeStr=boolean  PortDimensions=1
  MinusBtn : Inport  Port=2  OutDataTypeStr=boolean  PortDimensions=1
  Trigger : TriggerPort  VariantControl=Variant  PortDimensions=1
  Add : Sum  Inputs=++-
  Gain : Gain  Gain=Increment  ParamDataTypeStr=single  OutDataTypeStr=single
      settings: AttributesFormatString=%<Gain>
  Gain1 : Gain  Gain=Decrement  ParamDataTypeStr=single  OutDataTypeStr=single
      settings: AttributesFormatString=%<Gain>
  Saturation : Saturate  UpperLimit=MaxSetPoint  LowerLimit=MinSetPoint
      settings: AttributesFormatString=[%<LowerLimit> - %<UpperLimit>]
  Unit Delay : UnitDelay  InitialCondition=DefaultSetPoint  SampleTime=-1
  Setpoint : Outport  OutDataTypeStr=single  PortDimensions=1  InitialOutput=DefaultSetPoint
  wires:
  Gain/1 -> Add/2
  Gain1/1 -> Add/3
  PlusBtn/1 -> Gain/1
  MinusBtn/1 -> Gain1/1
  Unit Delay/1 -> Add/1
  Add/1 -> Saturation/1
  Saturation/1 -> Unit Delay/1, Setpoint/1

== system RespiratorCtrlLib/Outputs/Digital Write/Set on value changed ==
  In1 : Inport
  Enable : EnablePort
  MBED_DIG_OUT : mbedblockslib/Digital Write  Pin=2147483647  Direction=output
      settings: SourceProductName=Simulink Coder Support Package for BBC microbit Board  SourceProductBaseCode=MICROBIT
  wires:
  In1/1 -> MBED_DIG_OUT/1

== system RespiratorCtrlLib/Outputs/PWM Output/Set on value changed ==
  In1 : Inport
  Enable : EnablePort
  Data Type Conversion : DataTypeConversion
  MBED_PWM_OUT : mbedblockslib/PWM Output  Pin=2147483647  EnableInputFrequency=off  InitialFrequency=1000  InitialDutyCycle=0  NotificationType=None
      settings: SourceProductName=Simulink Coder Support Package for BBC microbit Board  SourceProductBaseCode=MICROBIT
  wires:
  Data Type Conversion/1 -> MBED_PWM_OUT/1
  In1/1 -> Data Type Conversion/1

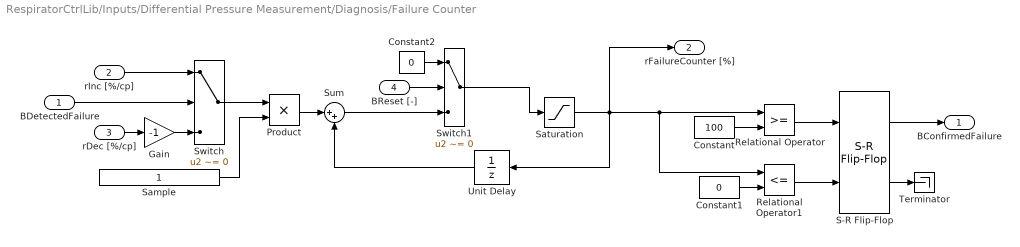
== system RespiratorCtrlLib/Inputs/Differential Pressure Measurement/Diagnosis/Failure Counter ==
  BDetectedFailure : Inport
  rInc [%/cp] : Inport  Port=2
  rDec [%/cp] : Inport  Port=3
  BReset [-] : Inport  Port=4
  Constant : Constant  Value=100
  Constant1 : Constant  Value=0
  Constant2 : Constant  Value=0
  Gain : Gain  Gain=-1
  Product : Product  RndMeth=Zero
  Relational Operator : RelationalOperator  OutDataTypeStr=boolean  RndMeth=Nearest
  Relational Operator1 : RelationalOperator  Operator=<=  OutDataTypeStr=boolean  RndMeth=Nearest
  S-R Flip-Flop : simulink_extras/Flip Flops/S-R Flip-Flop  initial_condition=0
  Sample : Constant
  Saturation : Saturate  UpperLimit=100  LowerLimit=0
      settings: AttributesFormatString=[%<LowerLimit>;%<UpperLimit>]
  Sum : Sum  Inputs=|++
  Switch : Switch  Criteria=u2 ~= 0
  Switch1 : Switch  Criteria=u2 ~= 0
  Terminator : Terminator
  Unit Delay : UnitDelay  SampleTime=-1
  BConfirmedFailure : Outport
  rFailureCounter [%] : Outport  Port=2
  wires:
  Product/1 -> Sum/1
  Sample/1 -> Product/2
  Gain/1 -> Switch/3
  Constant1/1 -> Relational Operator1/2
  Relational Operator1/1 -> S-R Flip-Flop/2
  Relational Operator/1 -> S-R Flip-Flop/1
  Constant/1 -> Relational Operator/2
  Saturation/1 -> Relational Operator1/1, Relational Operator/1, rFailureCounter [%]/1, Unit Delay/1
  Unit Delay/1 -> Sum/2
  S-R Flip-Flop/1 -> BConfirmedFailure/1
  Sum/1 -> Switch1/3
  Switch/1 -> Product/1
  rDec [%/cp]/1 -> Gain/1
  rInc [%/cp]/1 -> Switch/1
  BDetectedFailure/1 -> Switch/2
  S-R Flip-Flop/2 -> Terminator/1
  Constant2/1 -> Switch1/1
  BReset [-]/1 -> Switch1/2
  Switch1/1 -> Saturation/1
